simulink model "SB1_first_done"  (R2024b)
settings: Solver=FixedStepDiscrete  StartTime=0.0  StopTime=20  FixedStep=0.05  RelTol=1e-3
settings Model: Creator=admin  LastModifiedBy=admin

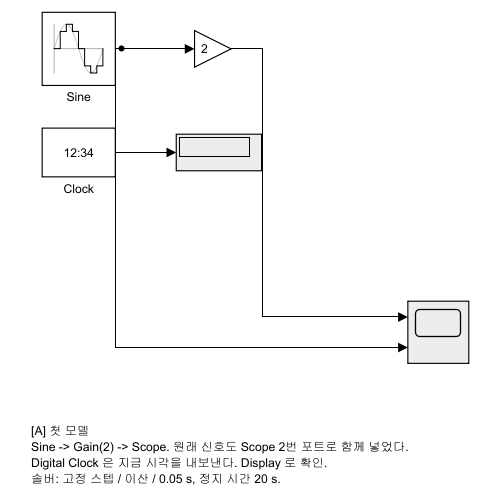
[thumbnail: Simulink's stored preview of the top-level diagram]
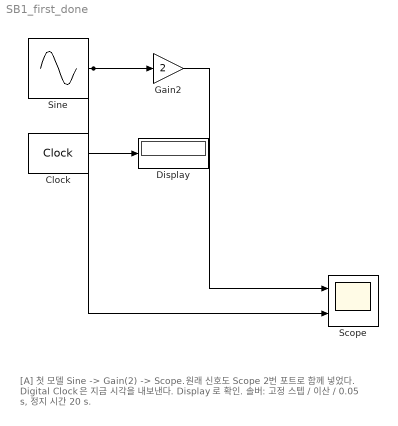
== system SB1_first_done ==
  note: [A] 첫 모델
      | Sine -> Gain(2) -> Scope. 원래 신호도 Scope 2번 포트로 함께 넣었다.
      | Digital Clock 은 지금 시각을 내보낸다. Display 로 확인.
      | 솔버: 고정 스텝 / 이산 / 0.05 s, 정지 시간 20 s.
  Clock : DigitalClock  SampleTime=0.05
  Display : Display
  Gain2 : Gain  Gain=2
  Scope : Scope  NumInputPorts=2
  Sine : Sin  SampleTime=0.05
  wires:
  Clock/1 -> Display/1
  Sine/1 -> Gain2/1, Scope/2
  Gain2/1 -> Scope/1
